simulink model "Two_Input_Events_2018a"  (R2018a)
settings: Solver=VariableStepAuto  StartTime=0.0  StopTime=40  RelTol=1e-3
settings Model: Creator=apple  LastModifiedBy=BEAR
settings DataIOCC: ReturnWorkspaceOutputs=on
settings SFSimCC: SimUseLocalCustomCode=on
settings RTWCC: RTWUseLocalCustomCode=on

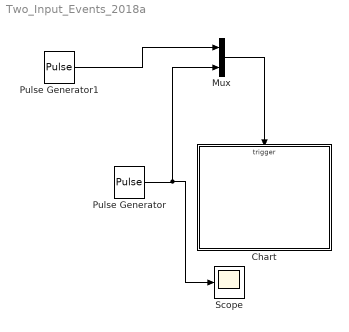
== system Two_Input_Events_2018a ==
  Chart : Stateflow chart  TreatAsAtomicUnit=on
  Mux : Mux  Inputs=2
  Pulse Generator : DiscretePulseGenerator  PulseType=Time based  Amplitude=3  Period=10  PulseWidth=50
  Pulse Generator1 : DiscretePulseGenerator  PulseType=Time based  Period=10  PulseWidth=50  PhaseDelay=5
  Scope : Scope
  wires:
  Pulse Generator/1 -> Mux/2, Scope/1
  Pulse Generator1/1 -> Mux/1
  Mux/1 -> Chart/Trigger

== stateflow chart Two_Input_Events_2018a/Chart ==
  settings: executeAtInitialization=1
  state On
    en:f("Entry_On");
    du:f("During_On");
    ex:f("Exit_On");
  state Off
    en:f("Entry_Off");
    du:f("During_Off");
    ex:f("Exit_Off");
  (default) -> On
  On -> Off : E_one/{f("E1")}
  Off -> On : E_two/{f("E2")}
  data: s function_input
  events: E_one input RISING_EDGE_EVENT; E_two input RISING_EDGE_EVENT
  function f(s):
    | function f(s)
    |   fprintf(s+"\n");
